simulink model "AXI_QPSK_Tx"  (R2023b)
settings: Solver=FixedStepAuto  StartTime=0.0  StopTime=10/Rb  RelTol=1e-3
PreLoadFcn:
  | Rb = 1000;   % 1kbit / s
  | Rsym = Rb/2;   % 2 bits per symbol
  | Rsymbol = Rb/2;
  | OSR = 32;
  | f_error = 120;
  | 
  | design_filters_tx
values from neighbouring files (symbols this model uses):
  CIC_fine_Tx = 2^-(CIC_right_shift - CIC_left_shift - CIC_shift_Tx)    [design_filters_tx.m]
  fCIC = fCICcomp * R_CIC    (= 25600000)    [design_filters_tx.m]
  fHB = fRRC * R_HB    (= 4000)    [design_filters_tx.m]
  R_CIC = 3200    [design_filters_tx.m]
  R_CICcomp = 2    [design_filters_tx.m]
  R_HB = 2    [design_filters_tx.m]
  R_RRC = 4    [design_filters_tx.m]
undefined symbols (not defined in the file or in its folder): AXI4, Lite
libraries: hdlBasic x309, hdlDSPIP x8, hdlsllib x2, vmcUtilities x1
(part 2 of 3)

== system AXI_QPSK_Tx/AXI_QPSK_Generator/M_AXIS_SYMBOL ==
  tdata_in : Inport
  tvalid_in : Inport  Port=2
  tlast_in : Inport  Port=3
  tready_in : Inport  Port=4
  m_symbol_axis_tdata : hdlBasic/Gateway Out  inherit_from_input=on  hdl_port=on  rows=1  columns=1  UseAsDAC=off  DACChannel='1'  interface=None  automatic_assignment=on  address_offset=hex2dec('00')  intf_name=''  intf_description=''  timing_constraint=None  locs_specified=off  LOCs={}  io_standard={}  XmcBlockStatus=1  maskContainerNames=group4  block_type=gatewayout  block_config=sysgen:gateway_out_config  block_width_w=590  block_height_w=620  block_width=620  block_height=750
  m_symbol_axis_tlast : hdlBasic/Gateway Out  inherit_from_input=off  hdl_port=on  rows=1  columns=1  UseAsDAC=off  DACChannel='1'  interface=None  automatic_assignment=on  address_offset=hex2dec('00')  intf_name=''  intf_description=''  timing_constraint=None  locs_specified=off  LOCs={}  io_standard={}  XmcBlockStatus=1  maskContainerNames=group4  block_type=gatewayout  block_config=sysgen:gateway_out_config  block_width_w=590  block_height_w=620  block_width=620  block_height=750
  m_symbol_axis_tready : hdlBasic/Gateway In  gui_display_data_type=Boolean  arith_type=Boolean  n_bits=16  bin_pt=14  preci_type=Single  exp_width=8  frac_width=24  rows=1  columns=1  quantization="Round  (unbiased: +/- Inf)"  overflow=Saturate  period=1/(fCIC)  UseAsADC=off  ADCChannel='1'  interface=None  automatic_assignment=on  address_offset=hex2dec('00')  intf_name=''  intf_description=''  default_value=0  timing_constraint=None  locs_specified=off  LOCs={}  io_standard={}  inherit_from_input=off  hdl_port=on  XmcBlockStatus=1  maskContainerNames=group4  block_type=gatewayin  block_config=sysgen:gateway_in_config  block_width_w=590  block_height_w=620  block_width=640  block_height=850
  m_symbol_axis_tvalid : hdlBasic/Gateway Out  inherit_from_input=off  hdl_port=on  rows=1  columns=1  UseAsDAC=off  DACChannel='1'  interface=None  automatic_assignment=on  address_offset=hex2dec('00')  intf_name=''  intf_description=''  timing_constraint=None  locs_specified=off  LOCs={}  io_standard={}  XmcBlockStatus=1  maskContainerNames=group4  block_type=gatewayout  block_config=sysgen:gateway_out_config  block_width_w=590  block_height_w=620  block_width=620  block_height=750
  tdata_out : Outport  VectorParamsAs1DForOutWhenUnconnected=off
  tvalid_out : Outport  Port=2  VectorParamsAs1DForOutWhenUnconnected=off
  tlast_out : Outport  Port=3  VectorParamsAs1DForOutWhenUnconnected=off
  tready_out : Outport  Port=4  VectorParamsAs1DForOutWhenUnconnected=off
  wires:
  tlast_in/1 -> m_symbol_axis_tlast/1
  m_symbol_axis_tlast/1 -> tlast_out/1
  m_symbol_axis_tready/1 -> tready_out/1
  tvalid_in/1 -> m_symbol_axis_tvalid/1
  m_symbol_axis_tvalid/1 -> tvalid_out/1
  tdata_in/1 -> m_symbol_axis_tdata/1
  m_symbol_axis_tdata/1 -> tdata_out/1
  tready_in/1 -> m_symbol_axis_tready/1

== system AXI_QPSK_Tx/AXI_QPSK_Generator/M_AXIS_TIME ==
  tdata_in : Inport
  tvalid_in : Inport  Port=2
  tlast_in : Inport  Port=3
  tready_in : Inport  Port=4
  m_time_axis_tdata : hdlBasic/Gateway Out  inherit_from_input=on  hdl_port=on  rows=1  columns=1  UseAsDAC=off  DACChannel='1'  interface=None  automatic_assignment=on  address_offset=hex2dec('00')  intf_name=''  intf_description=''  timing_constraint=None  locs_specified=off  LOCs={}  io_standard={}  XmcBlockStatus=1  maskContainerNames=group4  block_type=gatewayout  block_config=sysgen:gateway_out_config  block_width_w=590  block_height_w=620  block_width=620  block_height=750
  m_time_axis_tlast : hdlBasic/Gateway Out  inherit_from_input=off  hdl_port=on  rows=1  columns=1  UseAsDAC=off  DACChannel='1'  interface=None  automatic_assignment=on  address_offset=hex2dec('00')  intf_name=''  intf_description=''  timing_constraint=None  locs_specified=off  LOCs={}  io_standard={}  XmcBlockStatus=1  maskContainerNames=group4  block_type=gatewayout  block_config=sysgen:gateway_out_config  block_width_w=590  block_height_w=620  block_width=620  block_height=750
  m_time_axis_tready : hdlBasic/Gateway In  gui_display_data_type=Boolean  arith_type=Boolean  n_bits=16  bin_pt=14  preci_type=Single  exp_width=8  frac_width=24  rows=1  columns=1  quantization="Round  (unbiased: +/- Inf)"  overflow=Saturate  period=1/(fCIC)  UseAsADC=off  ADCChannel='1'  interface=None  automatic_assignment=on  address_offset=hex2dec('00')  intf_name=''  intf_description=''  default_value=0  timing_constraint=None  locs_specified=off  LOCs={}  io_standard={}  inherit_from_input=off  hdl_port=on  XmcBlockStatus=1  maskContainerNames=group4  block_type=gatewayin  block_config=sysgen:gateway_in_config  block_width_w=590  block_height_w=620  block_width=640  block_height=850
  m_time_axis_tvalid : hdlBasic/Gateway Out  inherit_from_input=off  hdl_port=on  rows=1  columns=1  UseAsDAC=off  DACChannel='1'  interface=None  automatic_assignment=on  address_offset=hex2dec('00')  intf_name=''  intf_description=''  timing_constraint=None  locs_specified=off  LOCs={}  io_standard={}  XmcBlockStatus=1  maskContainerNames=group4  block_type=gatewayout  block_config=sysgen:gateway_out_config  block_width_w=590  block_height_w=620  block_width=620  block_height=750
  tdata_out : Outport  VectorParamsAs1DForOutWhenUnconnected=off
  tvalid_out : Outport  Port=2  VectorParamsAs1DForOutWhenUnconnected=off
  tlast_out : Outport  Port=3  VectorParamsAs1DForOutWhenUnconnected=off
  tready_out : Outport  Port=4  VectorParamsAs1DForOutWhenUnconnected=off
  wires:
  tready_in/1 -> m_time_axis_tready/1
  m_time_axis_tdata/1 -> tdata_out/1
  tdata_in/1 -> m_time_axis_tdata/1
  m_time_axis_tvalid/1 -> tvalid_out/1
  tvalid_in/1 -> m_time_axis_tvalid/1
  m_time_axis_tready/1 -> tready_out/1
  m_time_axis_tlast/1 -> tlast_out/1
  tlast_in/1 -> m_time_axis_tlast/1

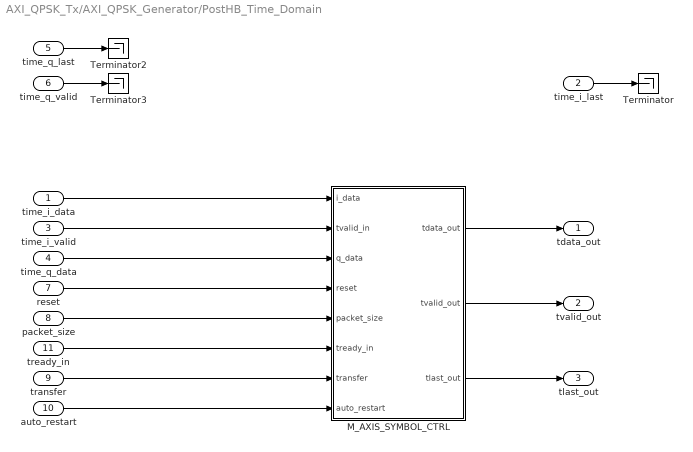
== system AXI_QPSK_Tx/AXI_QPSK_Generator/PostHB_Time_Domain ==
  time_i_data : Inport
  time_i_last : Inport  Port=2
  time_i_valid : Inport  Port=3
  time_q_data : Inport  Port=4
  time_q_last : Inport  Port=5
  time_q_valid : Inport  Port=6
  reset : Inport  Port=7
  packet_size : Inport  Port=8
  transfer : Inport  Port=9
  auto_restart : Inport  Port=10
  tready_in : Inport  Port=11
  M_AXIS_SYMBOL_CTRL : Subsystem
  Terminator : Terminator
  Terminator2 : Terminator
  Terminator3 : Terminator
  tdata_out : Outport  VectorParamsAs1DForOutWhenUnconnected=off
  tvalid_out : Outport  Port=2  VectorParamsAs1DForOutWhenUnconnected=off
  tlast_out : Outport  Port=3  VectorParamsAs1DForOutWhenUnconnected=off
  wires:
  auto_restart/1 -> M_AXIS_SYMBOL_CTRL/8(auto_restart)
  transfer/1 -> M_AXIS_SYMBOL_CTRL/7(transfer)
  M_AXIS_SYMBOL_CTRL/3(tlast_out) -> tlast_out/1
  M_AXIS_SYMBOL_CTRL/2(tvalid_out) -> tvalid_out/1
  M_AXIS_SYMBOL_CTRL/1(tdata_out) -> tdata_out/1
  tready_in/1 -> M_AXIS_SYMBOL_CTRL/6(tready_in)
  packet_size/1 -> M_AXIS_SYMBOL_CTRL/5(packet_size)
  reset/1 -> M_AXIS_SYMBOL_CTRL/4(reset)
  time_q_data/1 -> M_AXIS_SYMBOL_CTRL/3(q_data)
  time_i_valid/1 -> M_AXIS_SYMBOL_CTRL/2(tvalid_in)
  time_i_data/1 -> M_AXIS_SYMBOL_CTRL/1(i_data)
  time_q_valid/1 -> Terminator3/1
  time_q_last/1 -> Terminator2/1
  time_i_last/1 -> Terminator/1

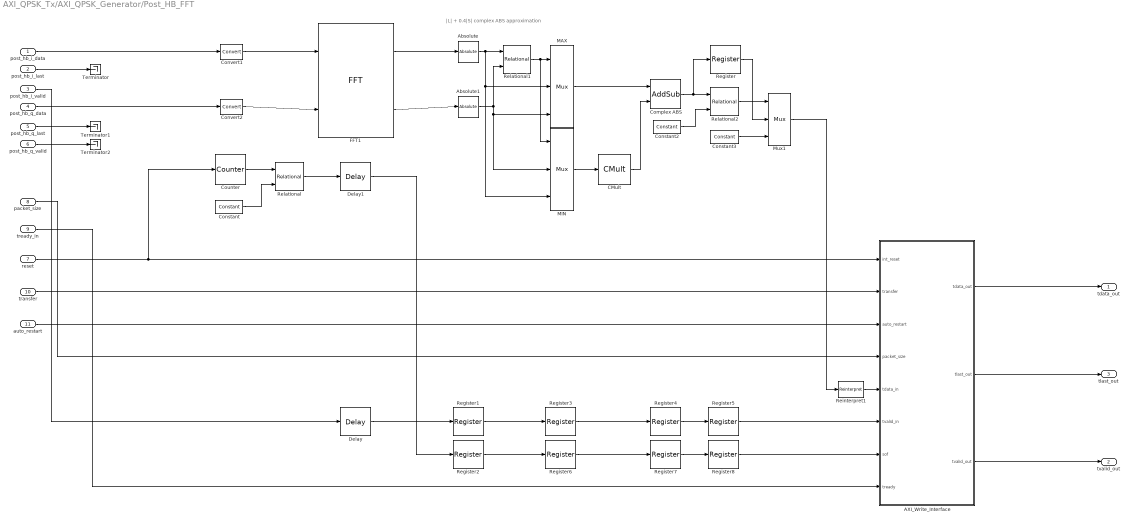
== system AXI_QPSK_Tx/AXI_QPSK_Generator/Post_HB_FFT ==
  note: |L| + 0.4|S| complex ABS approximation
  post_hb_i_data : Inport
  post_hb_i_last : Inport  Port=2
  post_hb_i_valid : Inport  Port=3
  post_hb_q_data : Inport  Port=4
  post_hb_q_last : Inport  Port=5
  post_hb_q_valid : Inport  Port=6
  reset : Inport  Port=7
  packet_size : Inport  Port=8
  tready_in : Inport  Port=9
  transfer : Inport  Port=10
  auto_restart : Inport  Port=11
  AXI_Write_Interface : Subsystem
  Absolute : hdlBasic/Absolute  precision=User Defined  arith_type=Unsigned  n_bits=32  bin_pt=31  quantization=Truncate  overflow=Wrap  en=off  latency=1  XmcBlockStatus=1  maskContainerNames=tabcontainer1  block_type=abs  block_config=sysgen:Abs_config
  Absolute1 : hdlBasic/Absolute  precision=User Defined  arith_type=Unsigned  n_bits=32  bin_pt=31  quantization=Truncate  overflow=Wrap  en=off  latency=1  XmcBlockStatus=1  maskContainerNames=tabcontainer1  block_type=abs  block_config=sysgen:Abs_config
  CMult : hdlBasic/CMult  const=0.4  gui_display_data_type=Fixed-point  const_n_bits=32  const_bin_pt=31  float_type=Single  exp_bits=8  fraction_bits=24  en=off  latency=0  precision=Full  arith_type=Unsigned  n_bits=15  bin_pt=15  quantization=Truncate  overflow=Wrap  use_behavioral_HDL=off  mem_type=Distributed RAM  pipeline=off  XmcBlockStatus=1  maskContainerNames=tabcontainer1  block_type=cmult  block_config=sysgen:CMult_config
      settings: infoedit=[]
  Complex ABS : hdlBasic/AddSub  mode=Addition  use_carryin=off  use_carryout=off  en=off  latency=1  precision=User Defined  arith_type=Unsigned  n_bits=32  bin_pt=31  quantization=Truncate  overflow=Wrap  use_behavioral_HDL=off  hw_selection=Fabric  pipelined=off  XmcBlockStatus=1  maskContainerNames=tabcontainer1  block_type=addsub  block_config=sysgen:Addsub_config
  Constant : hdlBasic/Constant  const=0  gui_display_data_type=Fixed-point  arith_type=Unsigned  n_bits=10  bin_pt=0  preci_type=Single  exp_width=8  frac_width=24  explicit_period=on  period=1/fHB  XmcBlockStatus=1  maskContainerNames=tabcontainer1  block_type=constant  block_config=sysgen:Constant_config
  Constant2 : hdlBasic/Constant  const=0  gui_display_data_type=Fixed-point  arith_type=Unsigned  n_bits=32  bin_pt=31  preci_type=Single  exp_width=8  frac_width=24  explicit_period=on  period=1/fHB  XmcBlockStatus=1  maskContainerNames=tabcontainer1  block_type=constant  block_config=sysgen:Constant_config
  Constant3 : hdlBasic/Constant  const=2^-31  gui_display_data_type=Fixed-point  arith_type=Unsigned  n_bits=32  bin_pt=31  preci_type=Single  exp_width=8  frac_width=24  explicit_period=on  period=1/fHB  XmcBlockStatus=1  maskContainerNames=tabcontainer1  block_type=constant  block_config=sysgen:Constant_config
  Convert1 : hdlBasic/Convert  gui_display_data_type=Fixed-point  arith_type="Signed  (2's comp)"  n_bits=32  bin_pt=31  float_type=Single  exp_bits=8  fraction_bits=24  quantization=Truncate  overflow=Wrap  en=off  latency=0  pipeline=off  XmcBlockStatus=1  maskContainerNames=group2  block_type=convert  block_config=sysgen:Convert_config  block_width=595  block_height=885
  Convert2 : hdlBasic/Convert  gui_display_data_type=Fixed-point  arith_type="Signed  (2's comp)"  n_bits=32  bin_pt=31  float_type=Single  exp_bits=8  fraction_bits=24  quantization=Truncate  overflow=Wrap  en=off  latency=0  pipeline=off  XmcBlockStatus=1  maskContainerNames=group2  block_type=convert  block_config=sysgen:Convert_config  block_width=595  block_height=885
  Counter : hdlBasic/Counter  cnt_type=Count limited  cnt_to=1023  operation=Up  start_count=0  cnt_by_val=1  arith_type=Unsigned  n_bits=10  bin_pt=0  load_pin=off  rst=on  en=off  explicit_period=Explicit  period=1/fHB  use_behavioral_HDL=off  implementation=Fabric  XmcBlockStatus=1  maskContainerNames=group1  block_type=counter  block_config=sysgen:Counter_config  block_width=531  block_height=1023
  Delay : hdlBasic/Delay  rst=off  en=off  latency=2204  reg_retiming=off  XmcBlockStatus=1  maskContainerNames=group1  block_type=delay  block_config=sysgen:Delay_config
  Delay1 : hdlBasic/Delay  rst=off  en=off  latency=2204  reg_retiming=off  XmcBlockStatus=1  maskContainerNames=group1  block_type=delay  block_config=sysgen:Delay_config
  FFT1 : hdlBasic/FFT  transform_length=1024  scale_result_by_fft_length=on  bit_reversed_order=on  optimizegoal=Performance  start_frame=off  simulation_type=fast_sim  simulation_model=sysgen:ForwardFFT_Macro  latency=1  XmcBlockStatus=1  maskContainerNames=group1  block_type=xfft_forward  block_config=sysgen:FFTMacro_config
  MAX : hdlBasic/Mux  inputs=2  en=off  latency=1  precision=Full  arith_type=Unsigned  n_bits=16  bin_pt=14  quantization=Truncate  overflow=Wrap  XmcBlockStatus=1  maskContainerNames=tabcontainer1  block_type=mux  block_config=sysgen:Mux_config
  MIN : hdlBasic/Mux  inputs=2  en=off  latency=1  precision=Full  arith_type=Unsigned  n_bits=16  bin_pt=14  quantization=Truncate  overflow=Wrap  XmcBlockStatus=1  maskContainerNames=tabcontainer1  block_type=mux  block_config=sysgen:Mux_config
  Mux1 : hdlBasic/Mux  inputs=2  en=off  latency=0  precision=Full  arith_type=Unsigned  n_bits=16  bin_pt=14  quantization=Truncate  overflow=Wrap  XmcBlockStatus=1  maskContainerNames=tabcontainer1  block_type=mux  block_config=sysgen:Mux_config
  Register{,1..8} (9 alike) : hdlBasic/Register  init=0  rst=off  en=off  XmcBlockStatus=1  maskContainerNames=tabcontainer1  block_type=register  block_config=sysgen:Register_config
  Reinterpret1 : hdlBasic/Reinterpret  force_arith_type=on  arith_type=Unsigned  force_bin_pt=on  bin_pt=0  XmcBlockStatus=1  maskContainerNames=group1  block_type=reinterpret  block_config=sysgen:Reinterpret_config
  Relational : hdlBasic/Relational  mode=a=b  op_type=Bool  en=off  latency=0  XmcBlockStatus=1  maskContainerNames=tabcontainer1  block_type=relational  block_config=sysgen:Relational_config
  Relational1 : hdlBasic/Relational  mode=a<b  op_type=Bool  en=off  latency=0  XmcBlockStatus=1  maskContainerNames=tabcontainer1  block_type=relational  block_config=sysgen:Relational_config
  Relational2 : hdlBasic/Relational  mode=a=b  op_type=Bool  en=off  latency=1  XmcBlockStatus=1  maskContainerNames=tabcontainer1  block_type=relational  block_config=sysgen:Relational_config
  Terminator : Terminator
  Terminator1 : Terminator
  Terminator2 : Terminator
  tdata_out : Outport  VectorParamsAs1DForOutWhenUnconnected=off
  tvalid_out : Outport  Port=2  VectorParamsAs1DForOutWhenUnconnected=off
  tlast_out : Outport  Port=3  VectorParamsAs1DForOutWhenUnconnected=off
  wires:
  post_hb_i_last/1 -> Terminator/1
  post_hb_q_last/1 -> Terminator1/1
  post_hb_q_valid/1 -> Terminator2/1
  AXI_Write_Interface/3(tvalid_out) -> tvalid_out/1
  AXI_Write_Interface/2(tlast_out) -> tlast_out/1
  packet_size/1 -> AXI_Write_Interface/4(packet_size)
  post_hb_i_valid/1 -> Delay/1
  Delay/1 -> Register1/1
  reset/1 -> Counter/1, AXI_Write_Interface/1(int_reset)
  FFT1/1 -> Absolute/1
  Relational1/1 -> MAX/1, MIN/1
  CMult/1 -> Complex ABS/2
  MAX/1 -> Complex ABS/1
  MIN/1 -> CMult/1
  Absolute1/1 -> MIN/2, MAX/3, Relational1/2
  Absolute/1 -> MAX/2, MIN/3, Relational1/1
  FFT1/2 -> Absolute1/1
  post_hb_i_data/1 -> Convert1/1
  AXI_Write_Interface/1(tdata_out) -> tdata_out/1
  transfer/1 -> AXI_Write_Interface/2(transfer)
  auto_restart/1 -> AXI_Write_Interface/3(auto_restart)
  Relational/1 -> Delay1/1
  tready_in/1 -> AXI_Write_Interface/8(tready)
  post_hb_q_data/1 -> Convert2/1
  Convert1/1 -> FFT1/1
  Convert2/1 -> FFT1/2
  Complex ABS/1 -> Register/1, Relational2/1
  Constant2/1 -> Relational2/2
  Relational2/1 -> Mux1/1
  Constant3/1 -> Mux1/3
  Register/1 -> Mux1/2
  Mux1/1 -> Reinterpret1/1
  Reinterpret1/1 -> AXI_Write_Interface/5(tdata_in)
  Counter/1 -> Relational/1
  Constant/1 -> Relational/2
  Delay1/1 -> Register2/1
  Register1/1 -> Register3/1
  Register2/1 -> Register6/1
  Register3/1 -> Register4/1
  Register4/1 -> Register5/1
  Register5/1 -> AXI_Write_Interface/6(tvalid_in)
  Register6/1 -> Register7/1
  Register7/1 -> Register8/1
  Register8/1 -> AXI_Write_Interface/7(sof)

== system AXI_QPSK_Tx/AXI_QPSK_Generator/QPSK_symbol_mapper ==
  note: Symbol rate =
      | 500sps
  Bit_pairs : Inport
  tlast_in : Inport  Port=2
  Reset : Inport  Port=3
  tready : Inport  Port=4
  Constant : hdlBasic/Constant  const=1.0  gui_display_data_type=Fixed-point  arith_type=Signed (2's comp)  n_bits=2  bin_pt=0  preci_type=Single  exp_width=8  frac_width=24  explicit_period=on  period=2/Rb  XmcBlockStatus=1  maskContainerNames=tabcontainer1  block_type=constant  block_config=sysgen:Constant_config
  Constant1 : hdlBasic/Constant  const=-1  gui_display_data_type=Fixed-point  arith_type=Signed (2's comp)  n_bits=2  bin_pt=0  preci_type=Single  exp_width=8  frac_width=24  explicit_period=on  period=2/Rb  XmcBlockStatus=1  maskContainerNames=tabcontainer1  block_type=constant  block_config=sysgen:Constant_config
  Constant2 : hdlBasic/Constant  const=1.0  gui_display_data_type=Fixed-point  arith_type=Signed (2's comp)  n_bits=2  bin_pt=0  preci_type=Single  exp_width=8  frac_width=24  explicit_period=on  period=2/Rb  XmcBlockStatus=1  maskContainerNames=tabcontainer1  block_type=constant  block_config=sysgen:Constant_config
  Constant3 : hdlBasic/Constant  const=-1  gui_display_data_type=Fixed-point  arith_type=Signed (2's comp)  n_bits=2  bin_pt=0  preci_type=Single  exp_width=8  frac_width=24  explicit_period=on  period=2/Rb  XmcBlockStatus=1  maskContainerNames=tabcontainer1  block_type=constant  block_config=sysgen:Constant_config
  Mux : hdlBasic/Mux  inputs=4  en=off  latency=0  precision=User Defined  arith_type="Signed  (2's comp)"  n_bits=2  bin_pt=0  quantization=Truncate  overflow=Wrap  XmcBlockStatus=1  maskContainerNames=tabcontainer1  block_type=mux  block_config=sysgen:Mux_config
  Mux1 : hdlBasic/Mux  inputs=4  en=off  latency=0  precision=User Defined  arith_type="Signed  (2's comp)"  n_bits=2  bin_pt=0  quantization=Truncate  overflow=Wrap  XmcBlockStatus=1  maskContainerNames=tabcontainer1  block_type=mux  block_config=sysgen:Mux_config
  Register : hdlBasic/Register  init=0  rst=on  en=on  XmcBlockStatus=1  maskContainerNames=tabcontainer1  block_type=register  block_config=sysgen:Register_config
  Register1 : hdlBasic/Register  init=0  rst=on  en=on  XmcBlockStatus=1  maskContainerNames=tabcontainer1  block_type=register  block_config=sysgen:Register_config
  Register2 : hdlBasic/Register  init=0  rst=on  en=on  XmcBlockStatus=1  maskContainerNames=tabcontainer1  block_type=register  block_config=sysgen:Register_config
  I_symbols : Outport  VectorParamsAs1DForOutWhenUnconnected=off
  Q_symbols : Outport  Port=2  VectorParamsAs1DForOutWhenUnconnected=off
  tlast_out : Outport  Port=3  VectorParamsAs1DForOutWhenUnconnected=off
  wires:
  Constant/1 -> Mux/3, Mux/2
  Constant3/1 -> Mux1/3, Mux1/5
  Register/1 -> I_symbols/1
  Bit_pairs/1 -> Mux/1, Mux1/1
  Constant2/1 -> Mux1/4, Mux1/2
  Mux/1 -> Register/1
  Mux1/1 -> Register1/1
  Constant1/1 -> Mux/5, Mux/4
  Register1/1 -> Q_symbols/1
  Reset/1 -> Register2/2, Register/2, Register1/2
  tready/1 -> Register/3, Register1/3, Register2/3
  tlast_in/1 -> Register2/1
  Register2/1 -> tlast_out/1

== system AXI_QPSK_Tx/AXI_QPSK_Generator/RF_Output ==
  rf_i_data : Inport
  rf_i_valid : Inport  Port=2
  rf_i_last : Inport  Port=3
  rf_q_data : Inport  Port=4
  rf_q_valid : Inport  Port=5
  rf_q_last : Inport  Port=6
  rf_ch_sel : Inport  Port=7
  Concat : hdlBasic/Concat  num_inputs=2  XmcBlockStatus=1  maskContainerNames=group1  block_type=concat  block_config=sysgen:Concat_config
  Logical1 : hdlBasic/Logical  logical_function=AND  inputs=2  en=off  latency=0  precision=Full  arith_type=Unsigned  n_bits=16  bin_pt=0  align_bp=on  overflow=[]  quantization=[]  XmcBlockStatus=1  maskContainerNames=tabcontainer1  block_type=logical  block_config=sysgen:Logical_config
  Logical2 : hdlBasic/Logical  logical_function=AND  inputs=2  en=off  latency=0  precision=Full  arith_type=Unsigned  n_bits=16  bin_pt=0  align_bp=on  overflow=[]  quantization=[]  XmcBlockStatus=1  maskContainerNames=tabcontainer1  block_type=logical  block_config=sysgen:Logical_config
  channel_selector : Subsystem
  ch0_out : Outport  VectorParamsAs1DForOutWhenUnconnected=off
  tvalid_in : Outport  Port=2  VectorParamsAs1DForOutWhenUnconnected=off
  tlast_in : Outport  Port=3  VectorParamsAs1DForOutWhenUnconnected=off
  ch1_out : Outport  Port=4  VectorParamsAs1DForOutWhenUnconnected=off
  ch2_out : Outport  Port=5  VectorParamsAs1DForOutWhenUnconnected=off
  ch3_out : Outport  Port=6  VectorParamsAs1DForOutWhenUnconnected=off
  wires:
  rf_q_data/1 -> Concat/1
  rf_i_last/1 -> Logical2/1
  rf_q_valid/1 -> Logical1/2
  rf_i_valid/1 -> Logical1/1
  Logical2/1 -> tlast_in/1
  rf_q_last/1 -> Logical2/2
  Logical1/1 -> tvalid_in/1
  rf_i_data/1 -> Concat/2
  channel_selector/1(ch0_out) -> ch0_out/1
  channel_selector/2(ch1_out) -> ch1_out/1
  channel_selector/3(ch2_out) -> ch2_out/1
  channel_selector/4(ch3_out) -> ch3_out/1
  Concat/1 -> channel_selector/2(data_in)
  rf_ch_sel/1 -> channel_selector/1(ch_sel)

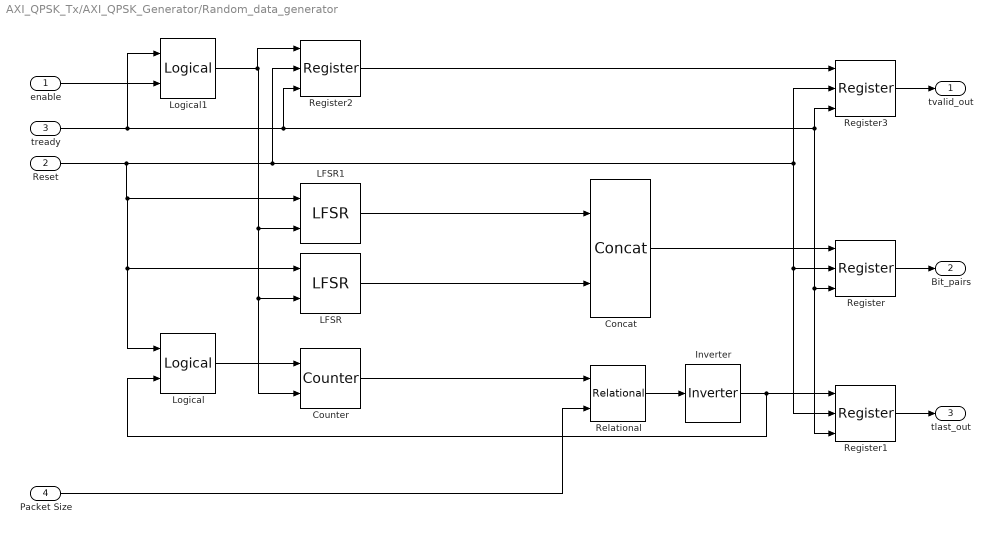
== system AXI_QPSK_Tx/AXI_QPSK_Generator/Random_data_generator ==
  enable : Inport
  Reset : Inport  Port=2
  tready : Inport  Port=3
  Packet Size : Inport  Port=4
  Concat : hdlBasic/Concat  num_inputs=2  XmcBlockStatus=1  maskContainerNames=group1  block_type=concat  block_config=sysgen:Concat_config
  Counter : hdlBasic/Counter  cnt_type=Free running  cnt_to=Inf  operation=Up  start_count=0  cnt_by_val=1  arith_type=Unsigned  n_bits=32  bin_pt=0  load_pin=off  rst=on  en=on  explicit_period=Explicit  period=2/Rb  use_behavioral_HDL=off  implementation=Fabric  XmcBlockStatus=1  maskContainerNames=group1  block_type=counter  block_config=sysgen:Counter_config  block_width=531  block_height=1023
  Inverter : hdlBasic/Inverter  en=off  latency=0  XmcBlockStatus=1  maskContainerNames=group2  block_type=inv  block_config=sysgen:Inverter_config
  LFSR : hdlBasic/LFSR  lfsr_type=Fibonacci  gate_type=XNOR  n_bits=10  maxpolynomial=on  polynomial='121'  rst_value='011'  rst=on  en=on  reloadable_seed=off  input_type=off  output_type=off  arith_type="Signed  (2's comp)"  bin_pt=4  explicit_period=on  period=2/Rb  XmcBlockStatus=1  maskContainerNames=tabcontainer1  block_type=lfsr  block_config=sysgen:LFSR_config
  LFSR1 : hdlBasic/LFSR  lfsr_type=Fibonacci  gate_type=XNOR  n_bits=10  maxpolynomial=on  polynomial='121'  rst_value='001'  rst=on  en=on  reloadable_seed=off  input_type=off  output_type=off  arith_type="Signed  (2's comp)"  bin_pt=4  explicit_period=on  period=2/Rb  XmcBlockStatus=1  maskContainerNames=tabcontainer1  block_type=lfsr  block_config=sysgen:LFSR_config
  Logical : hdlBasic/Logical  logical_function=OR  inputs=2  en=off  latency=0  precision=Full  arith_type=Unsigned  n_bits=16  bin_pt=0  align_bp=on  overflow=[]  quantization=[]  XmcBlockStatus=1  maskContainerNames=tabcontainer1  block_type=logical  block_config=sysgen:Logical_config
  Logical1 : hdlBasic/Logical  logical_function=AND  inputs=2  en=off  latency=0  precision=Full  arith_type=Unsigned  n_bits=16  bin_pt=0  align_bp=on  overflow=[]  quantization=[]  XmcBlockStatus=1  maskContainerNames=tabcontainer1  block_type=logical  block_config=sysgen:Logical_config
  Register{,1..3} (4 alike) : hdlBasic/Register  init=0  rst=on  en=on  XmcBlockStatus=1  maskContainerNames=tabcontainer1  block_type=register  block_config=sysgen:Register_config
  Relational : hdlBasic/Relational  mode=a<b  op_type=Bool  en=off  latency=0  XmcBlockStatus=1  maskContainerNames=tabcontainer1  block_type=relational  block_config=sysgen:Relational_config
  tvalid_out : Outport  VectorParamsAs1DForOutWhenUnconnected=off
  Bit_pairs : Outport  Port=2  VectorParamsAs1DForOutWhenUnconnected=off
  tlast_out : Outport  Port=3  VectorParamsAs1DForOutWhenUnconnected=off
  wires:
  tready/1 -> Logical1/1, Register1/3, Register/3, Register3/3, Register2/3
  Logical/1 -> Counter/1
  Concat/1 -> Register/1
  Register/1 -> Bit_pairs/1
  Reset/1 -> LFSR1/1, LFSR/1, Logical/1, Register3/2, Register1/2, Register/2, Register2/2
  Register1/1 -> tlast_out/1
  Relational/1 -> Inverter/1
  Inverter/1 -> Logical/2, Register1/1
  Packet Size/1 -> Relational/2
  enable/1 -> Logical1/2
  Logical1/1 -> Register2/1, LFSR1/2, LFSR/2, Counter/2
  Register3/1 -> tvalid_out/1
  LFSR/1 -> Concat/2
  LFSR1/1 -> Concat/1
  Counter/1 -> Relational/1
  Register2/1 -> Register3/1

== system AXI_QPSK_Tx/AXI_QPSK_Generator/Symbol_2_Output ==
  symbol_i_data : Inport
  symbol_i_last : Inport  Port=2
  symbol_i_valid : Inport  Port=3
  symbol_q_data : Inport  Port=4
  symbol_q_last : Inport  Port=5
  symbol_q_valid : Inport  Port=6
  reset : Inport  Port=7
  packet_size : Inport  Port=8
  transfer : Inport  Port=9
  auto_restart : Inport  Port=10
  tready_in : Inport  Port=11
  M_AXIS_SYMBOL_CTRL : Subsystem
  Terminator : Terminator
  Terminator2 : Terminator
  Terminator3 : Terminator
  tdata_out : Outport  VectorParamsAs1DForOutWhenUnconnected=off
  tvalid_out : Outport  Port=2  VectorParamsAs1DForOutWhenUnconnected=off
  tlast_out : Outport  Port=3  VectorParamsAs1DForOutWhenUnconnected=off
  wires:
  symbol_i_last/1 -> Terminator/1
  symbol_q_last/1 -> Terminator2/1
  symbol_q_valid/1 -> Terminator3/1
  symbol_i_data/1 -> M_AXIS_SYMBOL_CTRL/1(i_data)
  symbol_i_valid/1 -> M_AXIS_SYMBOL_CTRL/2(tvalid_in)
  symbol_q_data/1 -> M_AXIS_SYMBOL_CTRL/3(q_data)
  reset/1 -> M_AXIS_SYMBOL_CTRL/4(reset)
  packet_size/1 -> M_AXIS_SYMBOL_CTRL/5(packet_size)
  tready_in/1 -> M_AXIS_SYMBOL_CTRL/6(tready_in)
  M_AXIS_SYMBOL_CTRL/1(tdata_out) -> tdata_out/1
  M_AXIS_SYMBOL_CTRL/2(tvalid_out) -> tvalid_out/1
  M_AXIS_SYMBOL_CTRL/3(tlast_out) -> tlast_out/1
  transfer/1 -> M_AXIS_SYMBOL_CTRL/7(transfer)
  auto_restart/1 -> M_AXIS_SYMBOL_CTRL/8(auto_restart)

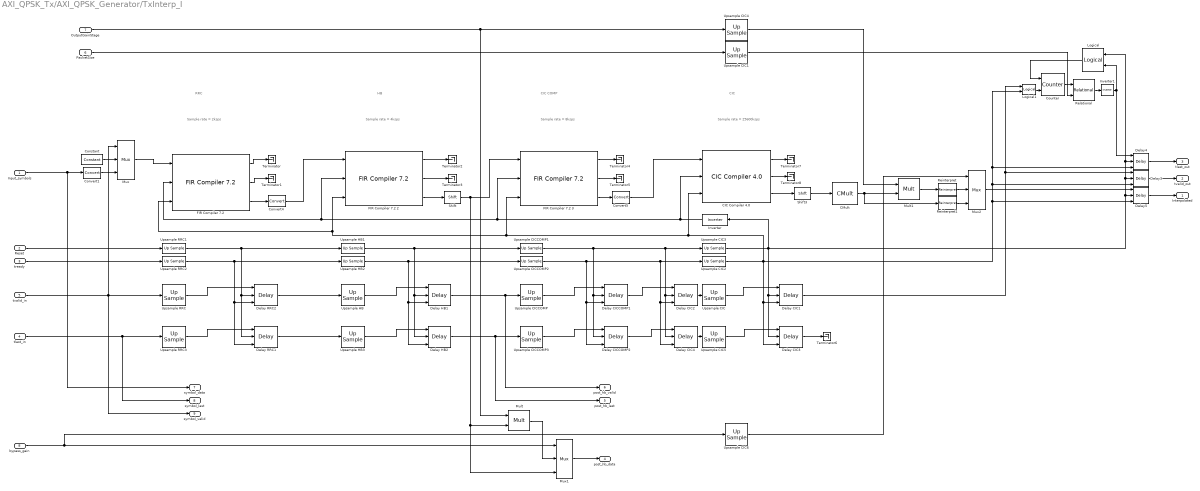
== system AXI_QPSK_Tx/AXI_QPSK_Generator/TxInterp_I ==
  note: HB
  note: RRC
  note: CIC COMP
  note: CIC
  note: Sample rate
      | = 2ksps
  note: Sample rate
      | = 4ksps
  note: Sample rate
      | = 8ksps
  note: Sample rate
      | = 25600ksps
  Input_symbols : Inport
  Reset : Inport  Port=2
  tready : Inport  Port=3
  tlast_in : Inport  Port=4
  tvalid_in : Inport  Port=5
  PacketSize : Inport  Port=6
  OutputGainStage : Inport  Port=7
  bypass_gain : Inport  Port=8
  "CIC Compiler 4.0 " : hdlDSPIP/CIC Compiler 4.0   filter_type=Interpolation  number_of_stages=5  differential_delay=1  number_of_channels=1  sample_rate_changes=Fixed  fixed_or_initial_rate=R_CIC  minimum_rate=3200  maximum_rate=3200  ratespecification=Maximum_Possible  sampleperiod=3200  hardwareoversamplingrate=1  quantization=Full_Precision  output_data_width=65  use_xtreme_dsp_slice=on  use_streaming_interface=on  has_aclken=on  has_aresetn=on  has_dout_tready=off  trim_axipin_name=on  gui_behaviour=Sysgen_GUI  input_data_width=18  ip_name=CIC Compiler  ip_version=4.0  dsptool_ready=true  wrapper_available=true  port_translation_map={ 'aclken' => 'en', 'aresetn' => 'rst' }  ipcore_xco_need_fpga_part=true  ipcore_fpga_part=[]  ipcore_verbose=false  XmcBlockStatus=1  maskContainerNames=tabcontainer1  block_type=cic_compiler_v4_0  block_config=sysgen:rodinimport_config
  CMult : hdlBasic/CMult  const=CIC_fine_Tx  gui_display_data_type=Fixed-point  const_n_bits=16  const_bin_pt=15  float_type=Single  exp_bits=8  fraction_bits=24  en=off  latency=0  precision=User Defined  arith_type="Signed  (2's comp)"  n_bits=16  bin_pt=15  quantization=Truncate  overflow=Wrap  use_behavioral_HDL=off  mem_type=Distributed RAM  pipeline=off  XmcBlockStatus=1  maskContainerNames=tabcontainer1  block_type=cmult  block_config=sysgen:CMult_config
      settings: infoedit=[]
  Constant : hdlBasic/Constant  const=0  gui_display_data_type=Fixed-point  arith_type=Signed (2's comp)  n_bits=16  bin_pt=0  preci_type=Single  exp_width=8  frac_width=24  explicit_period=on  period=2/Rb  XmcBlockStatus=1  maskContainerNames=tabcontainer1  block_type=constant  block_config=sysgen:Constant_config
  Convert1 : hdlBasic/Convert  gui_display_data_type=Fixed-point  arith_type=Signed (2's comp)  n_bits=16  bin_pt=0  float_type=Single  exp_bits=8  fraction_bits=24  quantization=Truncate  overflow=Wrap  en=off  latency=0  pipeline=off  XmcBlockStatus=1  maskContainerNames=group2  block_type=convert  block_config=sysgen:Convert_config  block_width=595  block_height=885
  Convert4 : hdlBasic/Convert  gui_display_data_type=Fixed-point  arith_type=Signed (2's comp)  n_bits=16  bin_pt=15  float_type=Single  exp_bits=8  fraction_bits=24  quantization=Truncate  overflow=Wrap  en=off  latency=0  pipeline=off  XmcBlockStatus=1  maskContainerNames=group2  block_type=convert  block_config=sysgen:Convert_config  block_width=595  block_height=885
  Convert5 : hdlBasic/Convert  gui_display_data_type=Fixed-point  arith_type=Signed (2's comp)  n_bits=16  bin_pt=15  float_type=Single  exp_bits=8  fraction_bits=24  quantization=Truncate  overflow=Wrap  en=off  latency=0  pipeline=off  XmcBlockStatus=1  maskContainerNames=group2  block_type=convert  block_config=sysgen:Convert_config  block_width=595  block_height=885
  Counter : hdlBasic/Counter  cnt_type=Free running  cnt_to=Inf  operation=Up  start_count=0  cnt_by_val=1  arith_type=Unsigned  n_bits=32  bin_pt=0  load_pin=off  rst=on  en=on  explicit_period=Explicit  period=1/fCIC  use_behavioral_HDL=off  implementation=Fabric  XmcBlockStatus=1  maskContainerNames=group1  block_type=counter  block_config=sysgen:Counter_config  block_width=531  block_height=1023
  Delay CIC1 : hdlBasic/Delay  rst=on  en=on  latency=3*8  reg_retiming=off  XmcBlockStatus=1  maskContainerNames=group1  block_type=delay  block_config=sysgen:Delay_config
  Delay CIC2 : hdlBasic/Delay  rst=on  en=on  latency=4  reg_retiming=off  XmcBlockStatus=1  maskContainerNames=group1  block_type=delay  block_config=sysgen:Delay_config
  Delay CIC3 : hdlBasic/Delay  rst=on  en=on  latency=3*8-1  reg_retiming=off  XmcBlockStatus=1  maskContainerNames=group1  block_type=delay  block_config=sysgen:Delay_config
  Delay CIC4 : hdlBasic/Delay  rst=on  en=on  latency=5  reg_retiming=off  XmcBlockStatus=1  maskContainerNames=group1  block_type=delay  block_config=sysgen:Delay_config
  Delay CICCOMP1 : hdlBasic/Delay  rst=on  en=on  latency=R_CICcomp*4  reg_retiming=off  XmcBlockStatus=1  maskContainerNames=group1  block_type=delay  block_config=sysgen:Delay_config
  Delay CICCOMP2 : hdlBasic/Delay  rst=on  en=on  latency=R_CICcomp*4+1  reg_retiming=off  XmcBlockStatus=1  maskContainerNames=group1  block_type=delay  block_config=sysgen:Delay_config
  Delay HB1 : hdlBasic/Delay  rst=on  en=on  latency=R_HB*2  reg_retiming=off  XmcBlockStatus=1  maskContainerNames=group1  block_type=delay  block_config=sysgen:Delay_config
  Delay HB2 : hdlBasic/Delay  rst=on  en=on  latency=R_HB*2+1  reg_retiming=off  XmcBlockStatus=1  maskContainerNames=group1  block_type=delay  block_config=sysgen:Delay_config
  Delay RRC1 : hdlBasic/Delay  rst=on  en=on  latency=3*R_RRC  reg_retiming=off  XmcBlockStatus=1  maskContainerNames=group1  block_type=delay  block_config=sysgen:Delay_config
  Delay RRC2 : hdlBasic/Delay  rst=on  en=on  latency=R_RRC*2+1  reg_retiming=off  XmcBlockStatus=1  maskContainerNames=group1  block_type=delay  block_config=sysgen:Delay_config
  Delay3 : hdlBasic/Delay  rst=on  en=on  latency=1  reg_retiming=off  XmcBlockStatus=1  maskContainerNames=group1  block_type=delay  block_config=sysgen:Delay_config
  Delay4 : hdlBasic/Delay  rst=on  en=on  latency=1  reg_retiming=off  XmcBlockStatus=1  maskContainerNames=group1  block_type=delay  block_config=sysgen:Delay_config
  Delay5 : hdlBasic/Delay  rst=on  en=on  latency=1  reg_retiming=off  XmcBlockStatus=1  maskContainerNames=group1  block_type=delay  block_config=sysgen:Delay_config
  "FIR Compiler 7.2 " : hdlDSPIP/FIR Compiler 7.2   coefficientvector=WRRC.Numerator  coefficient_sets=1  coefficient_reload=off  filter_type=Interpolation  rate_change_type=Integer  interpolation_rate=R_RRC  decimation_rate=1  zero_pack_factor=1  channel_sequence=Basic  number_channels=1  pattern_list='P4-0,P4-1,P4-2,P4-3,P4-4'  number_paths=1  ratespecification=Maximum_Possible  sampleperiod=1  hardwareoversamplingrate=1  coefficient_sign=Signed  quantization=Quantize_Only  coefficient_width=16  bestprecision=on  coefficient_fractional_bits=15  coefficient_structure=Inferred  output_rounding_mode=Full_Precision  output_width=31  filter_architecture=Systolic_Multiply_Accumulate  optimization_goal=Area  optimization_list='None'  data_buffer_type=Automatic  coefficient_buffer_type=Automatic  input_buffer_type=Automatic  output_buffer_type=Automatic  preference_for_other_storage=Automatic  multi_column_support=Automatic  columnconfig='7'  inter_column_pipe_length=4  data_has_tlast=Not_Required  m_data_has_tready=off  s_data_has_fifo=off  s_data_has_tuser=Not_Required  m_data_has_tuser=Not_Required  s_config_sync_mode=On_Vector  s_config_method=Single  num_reload_slots=1  has_aclken=on  has_aresetn=on  reset_data_vector=on  trim_axipin_name=on  simulation_type=hybrid_sim  simulation_model=sysgen:xfirv7_2_cmodel  data_path_portlist={ 's_axis_data_tdata', 'm_axis_data_tdata' }  passband_min=0.0  passband_max=0.5  stopband_min=0.5  stopband_max=1.0  filter_selection=1  gui_behaviour='Sysgen_GUI'  data_sign=Signed  data_width=16  data_fractional_bits=0  data_tuser_width=1  wrapper_available=true  ip_wrap_arbitrary_binary_point=true  ip_name=FIR Compiler  ip_version=7.2  dsptool_ready=true  ipcore_usecache=true  ipcore_useipmodelcache=true  port_translation_map={ 'aclken' => 'en', 'aresetn' => 'rst' }  run_core_at_system_period=true  ipcore_xco_need_fpga_part=true  ipcore_fpga_part=[]  XmcBlockStatus=1  maskContainerNames=tabcontainer1  block_type=fir_compiler_v7_2  block_config=sysgen:rodinimport_config  block_width=820  block_height=600
  FIR Compiler 7.2 2 : hdlDSPIP/FIR Compiler 7.2   coefficientvector=HB.Numerator  coefficient_sets=1  coefficient_reload=off  filter_type=Interpolation  rate_change_type=Integer  interpolation_rate=2  decimation_rate=1  zero_pack_factor=1  channel_sequence=Basic  number_channels=1  pattern_list='P4-0,P4-1,P4-2,P4-3,P4-4'  number_paths=1  ratespecification=Maximum_Possible  sampleperiod=1  hardwareoversamplingrate=1  coefficient_sign=Signed  quantization=Quantize_Only  coefficient_width=16  bestprecision=on  coefficient_fractional_bits=15  coefficient_structure=Inferred  output_rounding_mode=Full_Precision  output_width=32  filter_architecture=Systolic_Multiply_Accumulate  optimization_goal=Area  optimization_list='None'  data_buffer_type=Automatic  coefficient_buffer_type=Automatic  input_buffer_type=Automatic  output_buffer_type=Automatic  preference_for_other_storage=Automatic  multi_column_support=Automatic  columnconfig='6'  inter_column_pipe_length=4  data_has_tlast=Not_Required  m_data_has_tready=off  s_data_has_fifo=off  s_data_has_tuser=Not_Required  m_data_has_tuser=Not_Required  s_config_sync_mode=On_Vector  s_config_method=Single  num_reload_slots=1  has_aclken=on  has_aresetn=on  reset_data_vector=on  trim_axipin_name=on  simulation_type=hybrid_sim  simulation_model=sysgen:xfirv7_2_cmodel  data_path_portlist={ 's_axis_data_tdata', 'm_axis_data_tdata' }  passband_min=0.0  passband_max=0.5  stopband_min=0.5  stopband_max=1.0  filter_selection=1  gui_behaviour='Sysgen_GUI'  data_sign=Signed  data_width=16  data_fractional_bits=0  data_tuser_width=1  wrapper_available=true  ip_wrap_arbitrary_binary_point=true  ip_name=FIR Compiler  ip_version=7.2  dsptool_ready=true  ipcore_usecache=true  ipcore_useipmodelcache=true  port_translation_map={ 'aclken' => 'en', 'aresetn' => 'rst' }  run_core_at_system_period=true  ipcore_xco_need_fpga_part=true  ipcore_fpga_part=[]  XmcBlockStatus=1  maskContainerNames=tabcontainer1  block_type=fir_compiler_v7_2  block_config=sysgen:rodinimport_config  block_width=820  block_height=600
  FIR Compiler 7.2 3 : hdlDSPIP/FIR Compiler 7.2   coefficientvector=WComp.Numerator  coefficient_sets=1  coefficient_reload=off  filter_type=Interpolation  rate_change_type=Integer  interpolation_rate=R_CICcomp  decimation_rate=1  zero_pack_factor=1  channel_sequence=Basic  number_channels=1  pattern_list='P4-0,P4-1,P4-2,P4-3,P4-4'  number_paths=1  ratespecification=Maximum_Possible  sampleperiod=1  hardwareoversamplingrate=1  coefficient_sign=Signed  quantization=Quantize_Only  coefficient_width=16  bestprecision=on  coefficient_fractional_bits=15  coefficient_structure=Inferred  output_rounding_mode=Full_Precision  output_width=33  filter_architecture=Systolic_Multiply_Accumulate  optimization_goal=Area  optimization_list='None'  data_buffer_type=Automatic  coefficient_buffer_type=Automatic  input_buffer_type=Automatic  output_buffer_type=Automatic  preference_for_other_storage=Automatic  multi_column_support=Automatic  columnconfig='19'  inter_column_pipe_length=4  data_has_tlast=Not_Required  m_data_has_tready=off  s_data_has_fifo=off  s_data_has_tuser=Not_Required  m_data_has_tuser=Not_Required  s_config_sync_mode=On_Vector  s_config_method=Single  num_reload_slots=1  has_aclken=on  has_aresetn=on  reset_data_vector=on  trim_axipin_name=on  simulation_type=hybrid_sim  simulation_model=sysgen:xfirv7_2_cmodel  data_path_portlist={ 's_axis_data_tdata', 'm_axis_data_tdata' }  passband_min=0.0  passband_max=0.5  stopband_min=0.5  stopband_max=1.0  filter_selection=1  gui_behaviour='Sysgen_GUI'  data_sign=Signed  data_width=16  data_fractional_bits=0  data_tuser_width=1  wrapper_available=true  ip_wrap_arbitrary_binary_point=true  ip_name=FIR Compiler  ip_version=7.2  dsptool_ready=true  ipcore_usecache=true  ipcore_useipmodelcache=true  port_translation_map={ 'aclken' => 'en', 'aresetn' => 'rst' }  run_core_at_system_period=true  ipcore_xco_need_fpga_part=true  ipcore_fpga_part=[]  XmcBlockStatus=1  maskContainerNames=tabcontainer1  block_type=fir_compiler_v7_2  block_config=sysgen:rodinimport_config  block_width=820  block_height=600
  Inverter : hdlBasic/Inverter  en=off  latency=0  XmcBlockStatus=1  maskContainerNames=group2  block_type=inv  block_config=sysgen:Inverter_config
  Inverter1 : hdlBasic/Inverter  en=off  latency=0  XmcBlockStatus=1  maskContainerNames=group2  block_type=inv  block_config=sysgen:Inverter_config
  Logical : hdlBasic/Logical  logical_function=OR  inputs=2  en=off  latency=0  precision=Full  arith_type=Unsigned  n_bits=16  bin_pt=0  align_bp=on  overflow=[]  quantization=[]  XmcBlockStatus=1  maskContainerNames=tabcontainer1  block_type=logical  block_config=sysgen:Logical_config
  Logical1 : hdlBasic/Logical  logical_function=AND  inputs=2  en=off  latency=0  precision=Full  arith_type=Unsigned  n_bits=16  bin_pt=0  align_bp=on  overflow=[]  quantization=[]  XmcBlockStatus=1  maskContainerNames=tabcontainer1  block_type=logical  block_config=sysgen:Logical_config
  Mult : hdlBasic/Mult  precision=User Defined  arith_type="Signed  (2's comp)"  n_bits=16  bin_pt=15  quantization=Truncate  overflow=Wrap  en=off  latency=0  use_behavioral_HDL=off  opt=Speed  use_embedded=on  optimum_pipeline=off  pipeline=on  use_rpm=on  placement_style=Triangular  XmcBlockStatus=1  maskContainerNames=group1  block_type=mult  block_config=sysgen:Mult_config  block_width=598  block_height=876
  Mult1 : hdlBasic/Mult  precision=User Defined  arith_type="Signed  (2's comp)"  n_bits=16  bin_pt=15  quantization=Truncate  overflow=Wrap  en=off  latency=0  use_behavioral_HDL=off  opt=Speed  use_embedded=on  optimum_pipeline=off  pipeline=on  use_rpm=on  placement_style=Triangular  XmcBlockStatus=1  maskContainerNames=group1  block_type=mult  block_config=sysgen:Mult_config  block_width=598  block_height=876
  Mux : hdlBasic/Mux  inputs=2  en=off  latency=0  precision=Full  arith_type=Unsigned  n_bits=16  bin_pt=14  quantization=Truncate  overflow=Wrap  XmcBlockStatus=1  maskContainerNames=tabcontainer1  block_type=mux  block_config=sysgen:Mux_config
  Mux1 : hdlBasic/Mux  inputs=2  en=off  latency=0  precision=Full  arith_type=Unsigned  n_bits=16  bin_pt=14  quantization=Truncate  overflow=Wrap  XmcBlockStatus=1  maskContainerNames=tabcontainer1  block_type=mux  block_config=sysgen:Mux_config
  Mux2 : hdlBasic/Mux  inputs=2  en=off  latency=0  precision=Full  arith_type=Unsigned  n_bits=16  bin_pt=14  quantization=Truncate  overflow=Wrap  XmcBlockStatus=1  maskContainerNames=tabcontainer1  block_type=mux  block_config=sysgen:Mux_config
  Reinterpret : hdlBasic/Reinterpret  force_arith_type=on  arith_type=Unsigned  force_bin_pt=on  bin_pt=0  XmcBlockStatus=1  maskContainerNames=group1  block_type=reinterpret  block_config=sysgen:Reinterpret_config
  Reinterpret1 : hdlBasic/Reinterpret  force_arith_type=on  arith_type=Unsigned  force_bin_pt=on  bin_pt=0  XmcBlockStatus=1  maskContainerNames=group1  block_type=reinterpret  block_config=sysgen:Reinterpret_config
  Relational : hdlBasic/Relational  mode=a<b  op_type=Bool  en=off  latency=0  XmcBlockStatus=1  maskContainerNames=tabcontainer1  block_type=relational  block_config=sysgen:Relational_config
  Shift : hdlBasic/Shift  shift_dir=Left  shift_bits=1  en=off  latency=0  precision=User Defined  arith_type="Signed  (2's comp)"  n_bits=16  bin_pt=15  quantization=Truncate  overflow=Wrap  XmcBlockStatus=1  maskContainerNames=group2  block_type=shift  block_config=sysgen:Shift_config
  Shift3 : hdlBasic/Shift  shift_dir=Right  shift_bits=CIC_shift_Tx  en=off  latency=0  precision=User Defined  arith_type="Signed  (2's comp)"  n_bits=17  bin_pt=14  quantization=Truncate  overflow=Wrap  XmcBlockStatus=1  maskContainerNames=group2  block_type=shift  block_config=sysgen:Shift_config
  Terminator{,1..8} (9 alike) : Terminator
  Upsample CIC : hdlBasic/Up Sample  sample_ratio=R_CIC  copy_samples=on  en=off  latency=0  XmcBlockStatus=1  maskContainerNames=group1  block_type=usamp  block_config=sysgen:Upsample_config
  Upsample CIC1 : hdlBasic/Up Sample  sample_ratio=fCIC/(Rb/2)  copy_samples=on  en=off  latency=0  XmcBlockStatus=1  maskContainerNames=group1  block_type=usamp  block_config=sysgen:Upsample_config
  Upsample CIC2 : hdlBasic/Up Sample  sample_ratio=R_CIC  copy_samples=on  en=off  latency=0  XmcBlockStatus=1  maskContainerNames=group1  block_type=usamp  block_config=sysgen:Upsample_config
  Upsample CIC3 : hdlBasic/Up Sample  sample_ratio=R_CIC  copy_samples=on  en=off  latency=0  XmcBlockStatus=1  maskContainerNames=group1  block_type=usamp  block_config=sysgen:Upsample_config
  Upsample CIC4 : hdlBasic/Up Sample  sample_ratio=fCIC/fHB  copy_samples=on  en=off  latency=0  XmcBlockStatus=1  maskContainerNames=group1  block_type=usamp  block_config=sysgen:Upsample_config
  Upsample CIC5 : hdlBasic/Up Sample  sample_ratio=R_CIC  copy_samples=off  en=off  latency=0  XmcBlockStatus=1  maskContainerNames=group1  block_type=usamp  block_config=sysgen:Upsample_config
  Upsample CIC6 : hdlBasic/Up Sample  sample_ratio=fCIC/fHB  copy_samples=on  en=off  latency=0  XmcBlockStatus=1  maskContainerNames=group1  block_type=usamp  block_config=sysgen:Upsample_config
  Upsample CICCOMP : hdlBasic/Up Sample  sample_ratio=R_CICcomp  copy_samples=on  en=off  latency=0  XmcBlockStatus=1  maskContainerNames=group1  block_type=usamp  block_config=sysgen:Upsample_config
  Upsample CICCOMP1 : hdlBasic/Up Sample  sample_ratio=R_CICcomp  copy_samples=on  en=off  latency=0  XmcBlockStatus=1  maskContainerNames=group1  block_type=usamp  block_config=sysgen:Upsample_config
  Upsample CICCOMP2 : hdlBasic/Up Sample  sample_ratio=R_CICcomp  copy_samples=on  en=off  latency=0  XmcBlockStatus=1  maskContainerNames=group1  block_type=usamp  block_config=sysgen:Upsample_config
  Upsample CICCOMP3 : hdlBasic/Up Sample  sample_ratio=R_CICcomp  copy_samples=off  en=off  latency=0  XmcBlockStatus=1  maskContainerNames=group1  block_type=usamp  block_config=sysgen:Upsample_config
  Upsample HB : hdlBasic/Up Sample  sample_ratio=R_HB  copy_samples=on  en=off  latency=0  XmcBlockStatus=1  maskContainerNames=group1  block_type=usamp  block_config=sysgen:Upsample_config
  Upsample HB1 : hdlBasic/Up Sample  sample_ratio=R_HB  copy_samples=on  en=off  latency=0  XmcBlockStatus=1  maskContainerNames=group1  block_type=usamp  block_config=sysgen:Upsample_config
  Upsample HB2 : hdlBasic/Up Sample  sample_ratio=R_HB  copy_samples=on  en=off  latency=0  XmcBlockStatus=1  maskContainerNames=group1  block_type=usamp  block_config=sysgen:Upsample_config
  Upsample HB3 : hdlBasic/Up Sample  sample_ratio=R_HB  copy_samples=off  en=off  latency=0  XmcBlockStatus=1  maskContainerNames=group1  block_type=usamp  block_config=sysgen:Upsample_config
  Upsample RRC : hdlBasic/Up Sample  sample_ratio=R_RRC  copy_samples=on  en=off  latency=0  XmcBlockStatus=1  maskContainerNames=group1  block_type=usamp  block_config=sysgen:Upsample_config
  Upsample RRC1 : hdlBasic/Up Sample  sample_ratio=R_RRC  copy_samples=on  en=off  latency=0  XmcBlockStatus=1  maskContainerNames=group1  block_type=usamp  block_config=sysgen:Upsample_config
  Upsample RRC2 : hdlBasic/Up Sample  sample_ratio=R_RRC  copy_samples=on  en=off  latency=0  XmcBlockStatus=1  maskContainerNames=group1  block_type=usamp  block_config=sysgen:Upsample_config
  Upsample RRC3 : hdlBasic/Up Sample  sample_ratio=R_RRC  copy_samples=off  en=off  latency=0  XmcBlockStatus=1  maskContainerNames=group1  block_type=usamp  block_config=sysgen:Upsample_config
  Interpolated : Outport  VectorParamsAs1DForOutWhenUnconnected=off
  tvalid_out : Outport  Port=2  VectorParamsAs1DForOutWhenUnconnected=off
  tlast_out : Outport  Port=3  VectorParamsAs1DForOutWhenUnconnected=off
  post_hb_data : Outport  Port=4  VectorParamsAs1DForOutWhenUnconnected=off
  post_hb_last : Outport  Port=5  VectorParamsAs1DForOutWhenUnconnected=off
  post_hb_valid : Outport  Port=6  VectorParamsAs1DForOutWhenUnconnected=off
  symbol_data : Outport  Port=7  VectorParamsAs1DForOutWhenUnconnected=off
  symbol_last : Outport  Port=8  VectorParamsAs1DForOutWhenUnconnected=off
  symbol_valid : Outport  Port=9  VectorParamsAs1DForOutWhenUnconnected=off
  wires:
  bypass_gain/1 -> Mux1/1, Upsample CIC6/1
  Reinterpret1/1 -> Mux2/3
  Mux2/1 -> Delay5/1
  Reinterpret/1 -> Mux2/2
  OutputGainStage/1 -> Mult/1, Upsample CIC4/1
  CMult/1 -> Reinterpret1/1, Mult1/2
  Shift/1 -> Mux1/3, Mult/2, FIR Compiler 7.2 3/1
  Convert1/1 -> Mux/3
  Convert4/1 -> FIR Compiler 7.2 2/1
  "CIC Compiler 4.0 "/3 -> Shift3/1
  Logical1/1 -> Counter/2
  Delay5/1 -> Interpolated/1
  Delay3/1 -> tvalid_out/1
  Delay4/1 -> tlast_out/1
  Relational/1 -> Inverter1/1
  Inverter1/1 -> Logical/2, Delay4/1
  Logical/1 -> Counter/1
  Counter/1 -> Relational/1
  Upsample CIC1/1 -> Relational/2
  PacketSize/1 -> Upsample CIC1/1
  "FIR Compiler 7.2 "/1 -> Terminator/1
  "FIR Compiler 7.2 "/2 -> Terminator1/1
  Shift3/1 -> CMult/1
  "FIR Compiler 7.2 "/3 -> Convert4/1
  FIR Compiler 7.2 2/3 -> Shift/1
  FIR Compiler 7.2 2/2 -> Terminator3/1
  FIR Compiler 7.2 2/1 -> Terminator2/1
  FIR Compiler 7.2 3/3 -> Convert5/1
  FIR Compiler 7.2 3/1 -> Terminator4/1
  FIR Compiler 7.2 3/2 -> Terminator5/1
  "CIC Compiler 4.0 "/1 -> Terminator7/1
  Convert5/1 -> "CIC Compiler 4.0 "/1
  Reset/1 -> Upsample RRC1/1
  Upsample CIC/1 -> Delay CIC1/1
  "CIC Compiler 4.0 "/2 -> Terminator8/1
  Upsample CIC2/1 -> Delay CIC3/3, Delay CIC1/3, Logical1/2, Delay4/3, Delay3/3, Delay5/3, "FIR Compiler 7.2 "/3, FIR Compiler 7.2 2/3, FIR Compiler 7.2 3/3, "CIC Compiler 4.0 "/3
  Upsample CIC3/1 -> Delay CIC3/2, Delay CIC1/2, Delay5/2, Delay3/2, Logical/1, Delay4/2, Inverter/1
  tvalid_in/1 -> Upsample RRC/1, symbol_valid/1, Mux/1
  Delay RRC2/1 -> Upsample HB/1
  Upsample RRC/1 -> Delay RRC2/1
  Upsample HB/1 -> Delay HB1/1
  Upsample CICCOMP/1 -> Delay CICCOMP1/1
  Delay CIC1/1 -> Logical1/1, Delay3/1
  tready/1 -> Upsample RRC2/1
  Upsample CICCOMP3/1 -> Delay CICCOMP2/1
  Upsample HB3/1 -> Delay HB2/1
  Upsample RRC3/1 -> Delay RRC1/1
  Delay RRC1/1 -> Upsample HB3/1
  tlast_in/1 -> Upsample RRC3/1, symbol_last/1
  Upsample CICCOMP2/1 -> Delay CICCOMP2/3, Delay CICCOMP1/3, Delay CIC4/3, Delay CIC2/3, Upsample CIC2/1
  Upsample CICCOMP1/1 -> Delay CICCOMP2/2, Delay CICCOMP1/2, Delay CIC4/2, Delay CIC2/2, Upsample CIC3/1
  Upsample HB2/1 -> Delay HB2/3, Delay HB1/3, Upsample CICCOMP2/1
  Upsample HB1/1 -> Delay HB2/2, Delay HB1/2, Upsample CICCOMP1/1
  Upsample RRC2/1 -> Delay RRC1/3, Delay RRC2/3, Upsample HB2/1
  Upsample RRC1/1 -> Delay RRC1/2, Delay RRC2/2, Upsample HB1/1
  Upsample CIC5/1 -> Delay CIC3/1
  Inverter/1 -> FIR Compiler 7.2 3/2, "FIR Compiler 7.2 "/2, FIR Compiler 7.2 2/2, "CIC Compiler 4.0 "/2
  Delay CIC2/1 -> Upsample CIC/1
  Delay CICCOMP1/1 -> Delay CIC2/1
  Delay CIC4/1 -> Upsample CIC5/1
  Delay CICCOMP2/1 -> Delay CIC4/1
  Mux/1 -> "FIR Compiler 7.2 "/1
  Input_symbols/1 -> Convert1/1, symbol_data/1
  Constant/1 -> Mux/2
  Delay HB2/1 -> Upsample CICCOMP3/1, post_hb_last/1
  Delay HB1/1 -> post_hb_valid/1, Upsample CICCOMP/1
  Delay CIC3/1 -> Terminator6/1
  Mult1/1 -> Reinterpret/1
  Upsample CIC4/1 -> Mult1/1
  Mux1/1 -> post_hb_data/1
  Mult/1 -> Mux1/2
  Upsample CIC6/1 -> Mux2/1
